simulink model "upravljanje"  (R2018a)
settings: Solver=VariableStepAuto  StartTime=0.0  StopTime=10.0  RelTol=1e-3
values from neighbouring files (symbols this model uses):
  a21 = -4*k/(3*Mt)    (= -53333.3333333)    [HPS.m]
  a22 = -(Bp+b)/Mt    (= -13)    [HPS.m]
  a23 = Ap/Mt    (= 0.00065)    [HPS.m]
  a24 = 4*k/(3*Mt)    (= 53333.3333333)    [HPS.m]
  a25 = b/Mt    (= 10)    [HPS.m]
  a32 = -4*Be*Ap/Vt    (= -8450000000)    [HPS.m]
  a33 = -4*Be*(Ctp+Kc)/Vt    (= -2.6)    [HPS.m]
  a51 = 4*k/(3*m)    (= 26666.6666667)    [HPS.m]
  a52 = b/m    (= 5)    [HPS.m]
  a54 = -10*k/(3*m)    (= -66666.6666667)    [HPS.m]
  a55 = -(b+mu)/m    (= -5.001)    [HPS.m]
  a56 = 2*k/m    (= 40000)    [HPS.m]
  a74 = 4*k/m    (= 80000)    [HPS.m]
  a76 = -6*k/m    (= -120000)    [HPS.m]
settings Model: Creator=test4  LastModifiedBy=test4

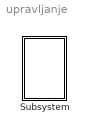
== system upravljanje ==
  Subsystem : Subsystem

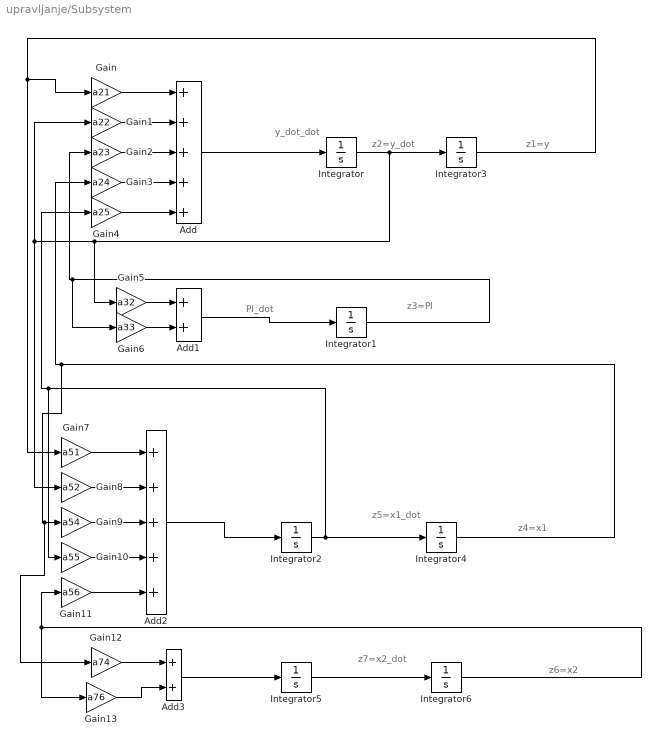
== system upravljanje/Subsystem ==
  note: z7=x2_dot
  note: z6=x2
  note: Pl_dot
  note: z5=x1_dot
  note: z4=x1
  note: y_dot_dot
  note: z3=Pl
  note: z1=y
  note: z2=y_dot
  Add : Sum  Inputs=+++++
  Add1 : Sum
  Add2 : Sum  Inputs=+++++
  Add3 : Sum
  Gain : Gain  Gain=a21
  Gain1 : Gain  Gain=a22
  Gain10 : Gain  Gain=a55
  Gain11 : Gain  Gain=a56
  Gain12 : Gain  Gain=a74
  Gain13 : Gain  Gain=a76
  Gain2 : Gain  Gain=a23
  Gain3 : Gain  Gain=a24
  Gain4 : Gain  Gain=a25
  Gain5 : Gain  Gain=a32
  Gain6 : Gain  Gain=a33
  Gain7 : Gain  Gain=a51
  Gain8 : Gain  Gain=a52
  Gain9 : Gain  Gain=a54
  Integrator{,1..6} (7 alike) : Integrator
  wires:
  Integrator/1 -> Gain5/1, Gain1/1, Gain8/1, Integrator3/1
  Integrator4/1 -> Gain12/1, Gain9/1, Gain3/1
  Gain13/1 -> Add3/2
  Gain4/1 -> Add/5
  Integrator5/1 -> Integrator6/1
  Integrator2/1 -> Integrator4/1, Gain10/1, Gain4/1
  Gain1/1 -> Add/2
  Add2/1 -> Integrator2/1
  Gain8/1 -> Add2/2
  Integrator6/1 -> Gain13/1, Gain11/1
  Add/1 -> Integrator/1
  Gain6/1 -> Add1/2
  Gain2/1 -> Add/3
  Integrator1/1 -> Gain6/1, Gain2/1
  Gain/1 -> Add/1
  Gain7/1 -> Add2/1
  Add3/1 -> Integrator5/1
  Gain10/1 -> Add2/4
  Add1/1 -> Integrator1/1
  Integrator3/1 -> Gain/1, Gain7/1
  Gain12/1 -> Add3/1
  Gain5/1 -> Add1/1
  Gain11/1 -> Add2/5
  Gain3/1 -> Add/4
  Gain9/1 -> Add2/3
